simulink model "AC_z"  (R2026a)
settings: Solver=VariableStepAuto
undefined symbols (not defined in the file or in its folder): Md, Mq, Mw, Uo, Zd, Zw
settings Model: Creator=devinbellll  LastModifiedBy=devinbellll

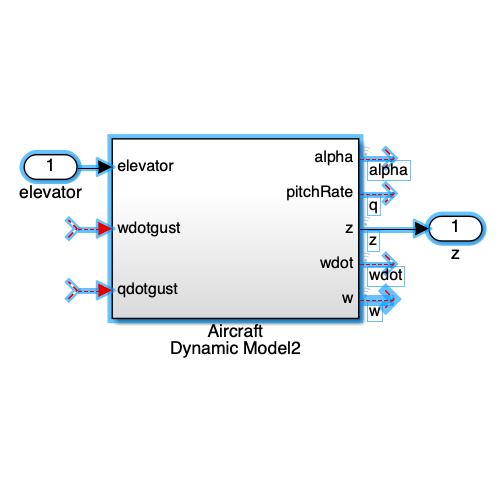
[thumbnail: Simulink's stored preview of the top-level diagram]
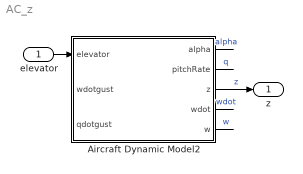
== system AC_z ==
  elevator : Inport
  Aircraft Dynamic Model2 : Subsystem
  z : Outport
  wires:
  elevator/1 -> Aircraft Dynamic Model2/1(elevator)
  Aircraft Dynamic Model2/4(wdot) -> ?  "wdot"
  Aircraft Dynamic Model2/3(z) -> z/1  "z"
  ? -> Aircraft Dynamic Model2/2(wdotgust)
  Aircraft Dynamic Model2/2(pitchRate) -> ?  "q"
  Aircraft Dynamic Model2/1(alpha) -> ?  "alpha"
  ? -> Aircraft Dynamic Model2/3(qdotgust)
  Aircraft Dynamic Model2/5(w) -> ?  "w"

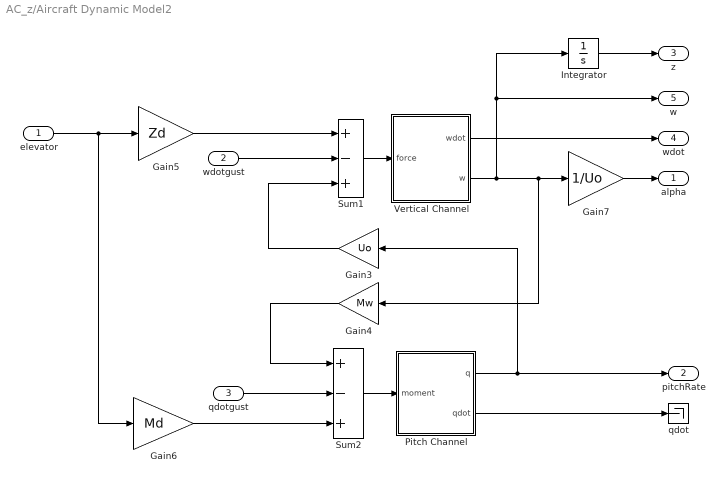
== system AC_z/Aircraft Dynamic Model2 ==
  elevator : Inport
  wdotgust : Inport  Port=2
  qdotgust : Inport  Port=3
  Gain3 : Gain  Gain=Uo  SaturateOnIntegerOverflow=on  OutDataTypeStr=Inherit: Same as input  ParamDataTypeStr=Inherit: Same as input
  Gain4 : Gain  Gain=Mw  SaturateOnIntegerOverflow=on  OutDataTypeStr=Inherit: Same as input  ParamDataTypeStr=Inherit: Same as input
  Gain5 : Gain  Gain=Zd  SaturateOnIntegerOverflow=on  OutDataTypeStr=Inherit: Same as input  ParamDataTypeStr=Inherit: Same as input
  Gain6 : Gain  Gain=Md  SaturateOnIntegerOverflow=on  OutDataTypeStr=Inherit: Same as input  ParamDataTypeStr=Inherit: Same as input
  Gain7 : Gain  Gain=1/Uo  SaturateOnIntegerOverflow=on  OutDataTypeStr=Inherit: Same as input  ParamDataTypeStr=Inherit: Same as input
  Integrator : Integrator
  Pitch Channel : Subsystem
  Sum1 : Sum  Inputs=+-+  InputSameDT=on  SaturateOnIntegerOverflow=on  OutDataTypeStr=Inherit: Same as first input
  Sum2 : Sum  Inputs=+-+  InputSameDT=on  SaturateOnIntegerOverflow=on  OutDataTypeStr=Inherit: Same as first input
  Vertical Channel : Subsystem
  qdot : Terminator
  alpha : Outport
  pitchRate : Outport  Port=2
  z : Outport  Port=3
  wdot : Outport  Port=4
  w : Outport  Port=5
  wires:
  Pitch Channel/1(q) -> Gain3/1, pitchRate/1
  Vertical Channel/2(w) -> Integrator/1, w/1, Gain7/1, Gain4/1
  Sum1/1 -> Vertical Channel/1(force)
  Gain6/1 -> Sum2/3
  Gain5/1 -> Sum1/1
  qdotgust/1 -> Sum2/2
  Sum2/1 -> Pitch Channel/1(moment)
  wdotgust/1 -> Sum1/2
  elevator/1 -> Gain6/1, Gain5/1
  Gain7/1 -> alpha/1
  Gain3/1 -> Sum1/3
  Gain4/1 -> Sum2/1
  Vertical Channel/1(wdot) -> wdot/1
  Pitch Channel/2(qdot) -> qdot/1
  Integrator/1 -> z/1

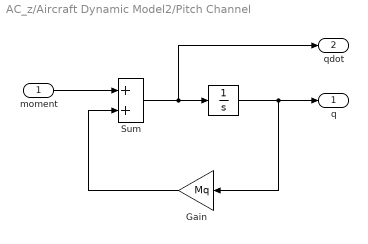
== system AC_z/Aircraft Dynamic Model2/Pitch Channel ==
  moment : Inport
  " " : Integrator
  Gain : Gain  Gain=Mq  SaturateOnIntegerOverflow=on  OutDataTypeStr=Inherit: Same as input  ParamDataTypeStr=Inherit: Same as input
  Sum : Sum  InputSameDT=on  SaturateOnIntegerOverflow=on  OutDataTypeStr=Inherit: Same as first input
  q : Outport
  qdot : Outport  Port=2
  wires:
  moment/1 -> Sum/1
  Gain/1 -> Sum/2
  " "/1 -> q/1, Gain/1
  Sum/1 -> qdot/1, " "/1

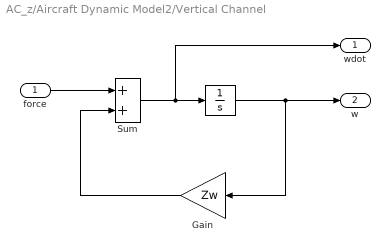
== system AC_z/Aircraft Dynamic Model2/Vertical Channel ==
  force : Inport
  " " : Integrator
  Gain : Gain  Gain=Zw  SaturateOnIntegerOverflow=on  OutDataTypeStr=Inherit: Same as input  ParamDataTypeStr=Inherit: Same as input
  Sum : Sum  InputSameDT=on  SaturateOnIntegerOverflow=on  OutDataTypeStr=Inherit: Same as first input
  wdot : Outport
  w : Outport  Port=2
  wires:
  Sum/1 -> wdot/1, " "/1
  " "/1 -> w/1, Gain/1
  Gain/1 -> Sum/2
  force/1 -> Sum/1
